simulink library "REC_lib"  (R2015a)
settings: Solver=ode45  StartTime=0.0  StopTime=10.0  RelTol=1e-3
undefined symbols (not defined in the file): REC
libraries: simulink x1, aerolibatmos2 x1
settings Model: Creator=Andrew  LastModifiedBy=Andrew

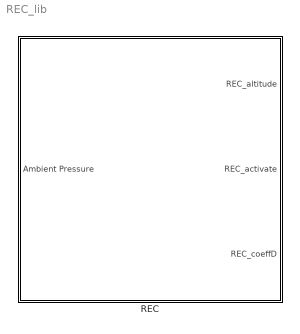
== system REC_lib ==
  REC : Subsystem

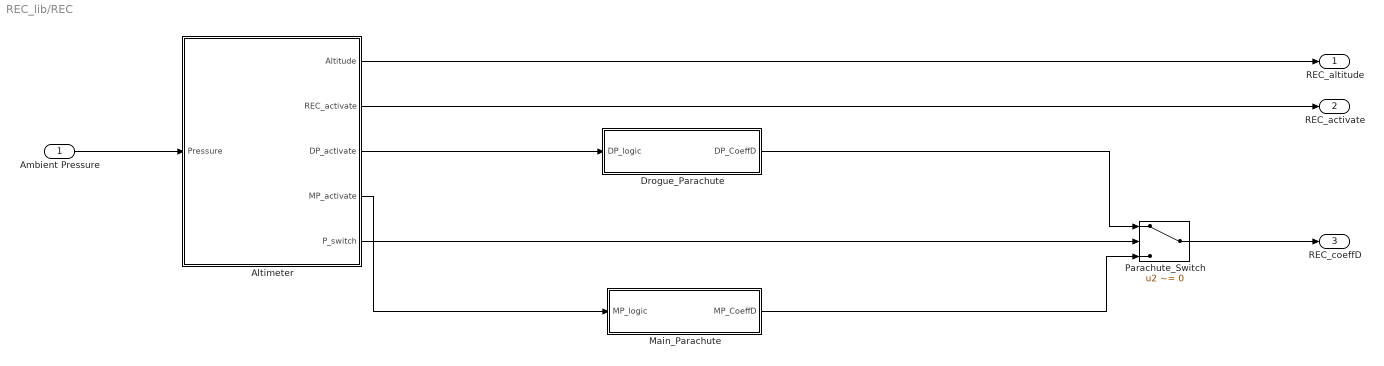
== system REC_lib/REC ==
  Ambient Pressure : Inport
  Altimeter : Subsystem
  Drogue_Parachute : Subsystem
  Main_Parachute : Subsystem
  Parachute_Switch : Switch  Criteria=u2 ~= 0
  REC_altitude : Outport
  REC_activate : Outport  Port=2
  REC_coeffD : Outport  Port=3
  wires:
  Altimeter/4(MP_activate) -> Main_Parachute/1(MP_logic)
  Altimeter/3(DP_activate) -> Drogue_Parachute/1(DP_logic)
  Ambient Pressure/1 -> Altimeter/1(Pressure)
  Altimeter/1(Altitude) -> REC_altitude/1
  Drogue_Parachute/1(DP_CoeffD) -> Parachute_Switch/1
  Main_Parachute/1(MP_CoeffD) -> Parachute_Switch/3
  Altimeter/2(REC_activate) -> REC_activate/1
  Parachute_Switch/1 -> REC_coeffD/1
  Altimeter/5(P_switch) -> Parachute_Switch/2

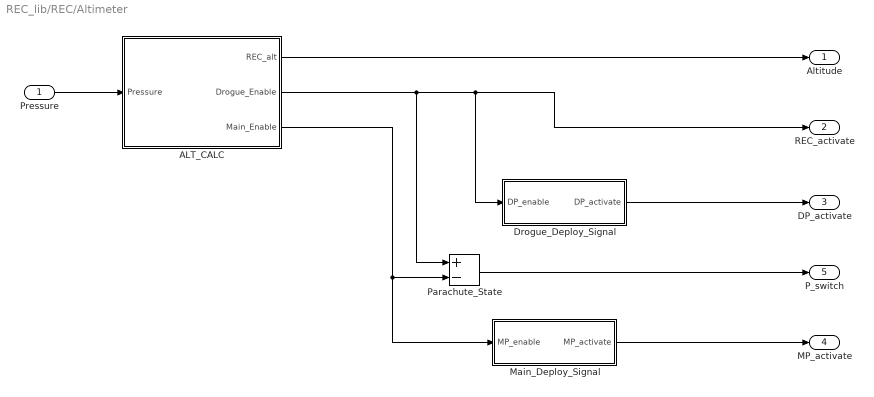
== system REC_lib/REC/Altimeter ==
  Pressure : Inport
  ALT_CALC : Subsystem
  Drogue_Deploy_Signal : Subsystem  TreatAsAtomicUnit=on
  Main_Deploy_Signal : Subsystem  TreatAsAtomicUnit=on
  Parachute_State : Sum  Inputs=+-
  Altitude : Outport
  REC_activate : Outport  Port=2
  DP_activate : Outport  Port=3
  MP_activate : Outport  Port=4
  P_switch : Outport  Port=5
  wires:
  Pressure/1 -> ALT_CALC/1(Pressure)
  ALT_CALC/1(REC_alt) -> Altitude/1
  ALT_CALC/2(Drogue_Enable) -> Parachute_State/1, Drogue_Deploy_Signal/1(DP_enable), REC_activate/1
  ALT_CALC/3(Main_Enable) -> Parachute_State/2, Main_Deploy_Signal/1(MP_enable)
  Drogue_Deploy_Signal/1(DP_activate) -> DP_activate/1
  Main_Deploy_Signal/1(MP_activate) -> MP_activate/1
  Parachute_State/1 -> P_switch/1

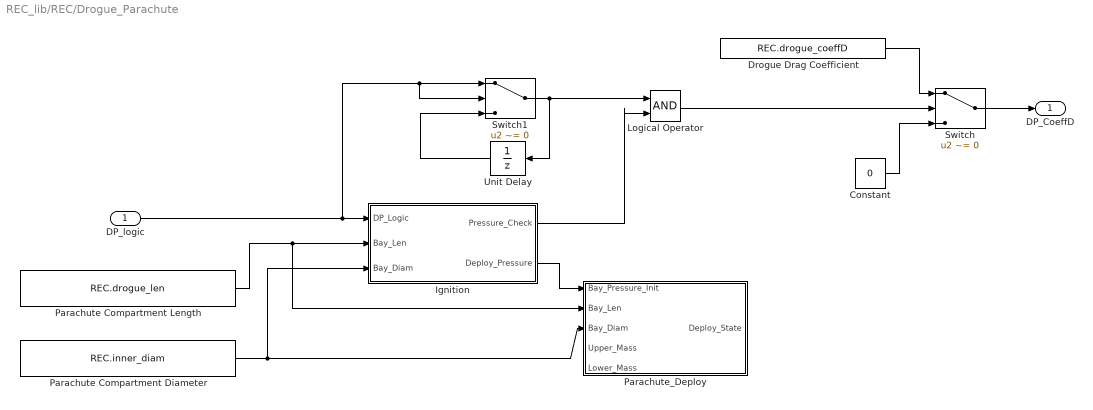
== system REC_lib/REC/Drogue_Parachute ==
  DP_logic : Inport
  Constant : Constant  Value=0
  Drogue Drag Coefficient : FromWorkspace  VariableName=REC.drogue_coeffD  SampleTime=0
  Ignition : Subsystem
  Logical Operator : Logic  AllPortsSameDT=off  OutDataTypeStr=boolean
  Parachute Compartment Diameter : FromWorkspace  VariableName=REC.inner_diam  SampleTime=0
  Parachute Compartment Length : FromWorkspace  VariableName=REC.drogue_len  SampleTime=0
  Parachute_Deploy : Subsystem
  Switch : Switch  Criteria=u2 ~= 0
  Switch1 : Switch  Criteria=u2 ~= 0
  Unit Delay : UnitDelay  SampleTime=-1
  DP_CoeffD : Outport
  wires:
  Switch/1 -> DP_CoeffD/1
  Drogue Drag Coefficient/1 -> Switch/1
  Constant/1 -> Switch/3
  DP_logic/1 -> Switch1/1, Switch1/2, Ignition/1(DP_Logic)
  Unit Delay/1 -> Switch1/3
  Switch1/1 -> Logical Operator/1, Unit Delay/1
  Logical Operator/1 -> Switch/2
  Parachute Compartment Diameter/1 -> Parachute_Deploy/3(Bay_Diam), Ignition/3(Bay_Diam)
  Ignition/1(Pressure_Check) -> Logical Operator/2
  Ignition/2(Deploy_Pressure) -> Parachute_Deploy/1(Bay_Pressure_Init)
  Parachute Compartment Length/1 -> Ignition/2(Bay_Len), Parachute_Deploy/2(Bay_Len)

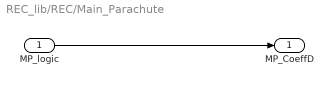
== system REC_lib/REC/Main_Parachute ==
  MP_logic : Inport
  MP_CoeffD : Outport
  wires:
  MP_logic/1 -> MP_CoeffD/1

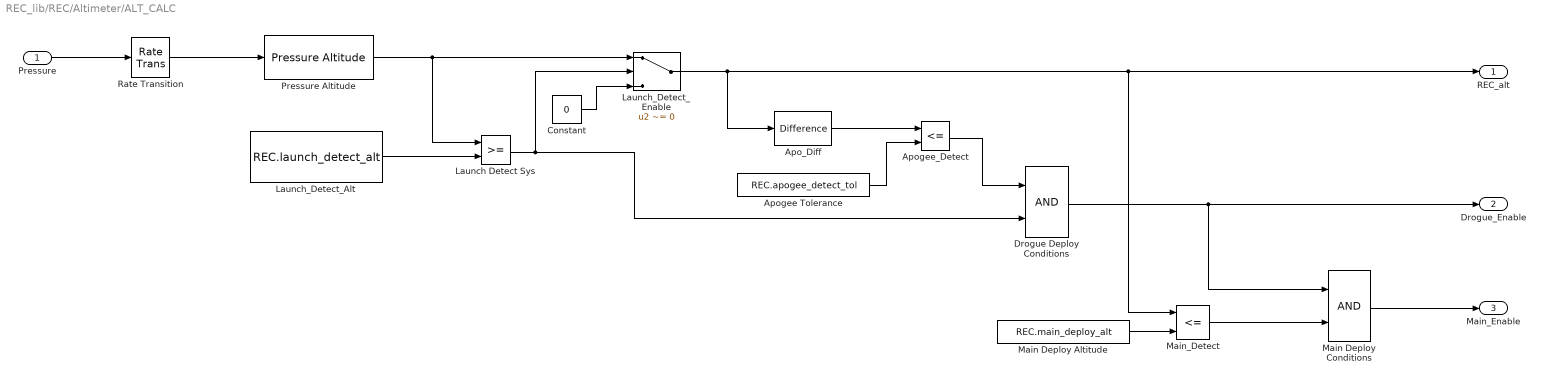
== system REC_lib/REC/Altimeter/ALT_CALC ==
  Pressure : Inport
  Apo_Diff : simulink/Discrete/Difference  ICPrevInput=0.0  InputProcessing=Inherited  OutMin=[]  OutMax=[]  OutDataType=fixdt(1, 16)  OutScaling=2^-10  DoSatur=off
  Apogee Tolerance : FromWorkspace  VariableName=REC.apogee_detect_tol  SampleTime=0
  Apogee_Detect : RelationalOperator  Operator=<=  OutDataTypeStr=boolean
  Constant : Constant  Value=0
  Drogue Deploy Conditions : Logic  AllPortsSameDT=off  OutDataTypeStr=boolean
  Launch Detect Sys : RelationalOperator  OutDataTypeStr=boolean
  Launch_Detect_Alt : FromWorkspace  VariableName=REC.launch_detect_alt  SampleTime=0
  Launch_Detect_Enable : Switch  Criteria=u2 ~= 0
  Main Deploy Altitude : FromWorkspace  VariableName=REC.main_deploy_alt  SampleTime=0
  Main Deploy Conditions : Logic  AllPortsSameDT=off  OutDataTypeStr=boolean
  Main_Detect : RelationalOperator  Operator=<=  OutDataTypeStr=boolean
  Pressure Altitude : aerolibatmos2/Pressure Altitude  units=English  action=Warning
  Rate Transition : RateTransition  OutPortSampleTime=REC.altimeter_sample_time
  REC_alt : Outport
  Drogue_Enable : Outport  Port=2
  Main_Enable : Outport  Port=3
  wires:
  Main Deploy Altitude/1 -> Main_Detect/2
  Apo_Diff/1 -> Apogee_Detect/1
  Pressure/1 -> Rate Transition/1
  Rate Transition/1 -> Pressure Altitude/1
  Apogee Tolerance/1 -> Apogee_Detect/2
  Launch Detect Sys/1 -> Drogue Deploy Conditions/2, Launch_Detect_Enable/2
  Main Deploy Conditions/1 -> Main_Enable/1
  Launch_Detect_Alt/1 -> Launch Detect Sys/2
  Apogee_Detect/1 -> Drogue Deploy Conditions/1
  Constant/1 -> Launch_Detect_Enable/3
  Pressure Altitude/1 -> Launch_Detect_Enable/1, Launch Detect Sys/1
  Launch_Detect_Enable/1 -> Apo_Diff/1, REC_alt/1, Main_Detect/1
  Main_Detect/1 -> Main Deploy Conditions/2
  Drogue Deploy Conditions/1 -> Drogue_Enable/1, Main Deploy Conditions/1

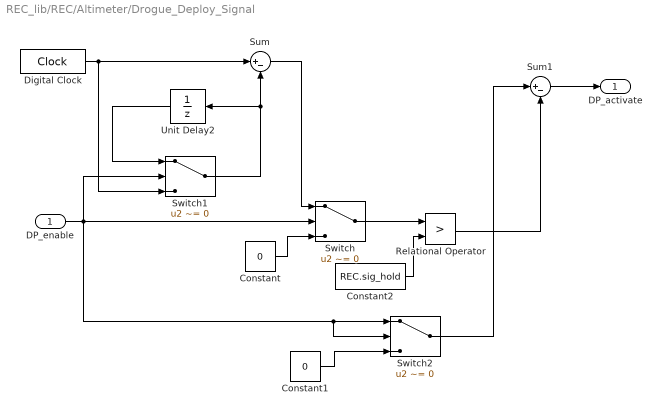
== system REC_lib/REC/Altimeter/Drogue_Deploy_Signal ==
  DP_enable : Inport
  Constant : Constant  Value=0
  Constant1 : Constant  Value=0
  Constant2 : Constant  Value=REC.sig_hold
  Digital Clock : DigitalClock  SampleTime=0.0025
  Relational Operator : RelationalOperator  Operator=>  OutDataTypeStr=boolean
  Sum : Sum  Inputs=|+-
  Sum1 : Sum  Inputs=|+-
  Switch : Switch  Criteria=u2 ~= 0
  Switch1 : Switch  Criteria=u2 ~= 0
  Switch2 : Switch  Criteria=u2 ~= 0
  Unit Delay2 : UnitDelay  SampleTime=-1
  DP_activate : Outport
  wires:
  Constant/1 -> Switch/3
  Digital Clock/1 -> Sum/1, Switch1/3
  Sum/1 -> Switch/1
  Switch/1 -> Relational Operator/1
  Switch1/1 -> Unit Delay2/1, Sum/2
  Unit Delay2/1 -> Switch1/1
  DP_enable/1 -> Switch2/1, Switch2/2, Switch1/2, Switch/2
  Constant1/1 -> Switch2/3
  Sum1/1 -> DP_activate/1
  Switch2/1 -> Sum1/1
  Relational Operator/1 -> Sum1/2
  Constant2/1 -> Relational Operator/2

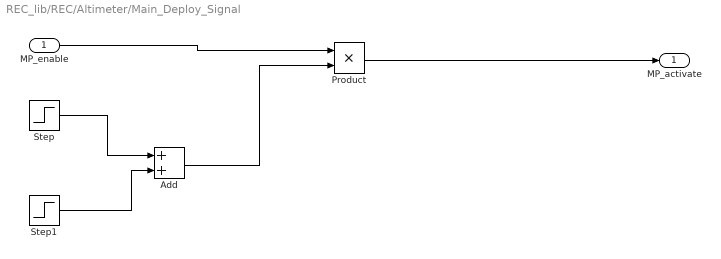
== system REC_lib/REC/Altimeter/Main_Deploy_Signal ==
  MP_enable : Inport
  Add : Sum
  Product : Product
  Step : Step  Time=0  SampleTime=0
  Step1 : Step  After=-1  SampleTime=0
  MP_activate : Outport
  wires:
  Product/1 -> MP_activate/1
  MP_enable/1 -> Product/1
  Step/1 -> Add/1
  Step1/1 -> Add/2
  Add/1 -> Product/2

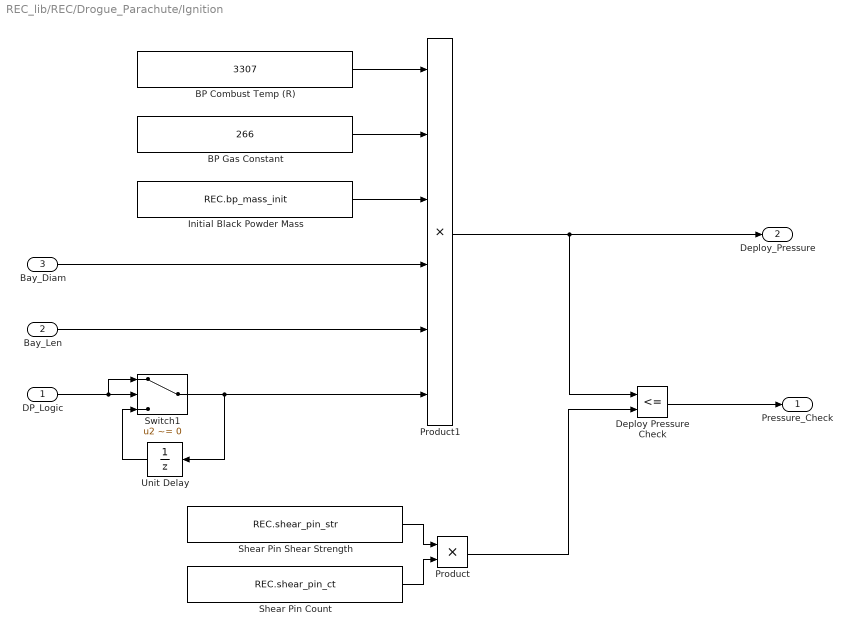
== system REC_lib/REC/Drogue_Parachute/Ignition ==
  DP_Logic : Inport
  Bay_Len : Inport  Port=2
  Bay_Diam : Inport  Port=3
  BP Combust Temp (R) : FromWorkspace  VariableName=3307  SampleTime=0
  BP Gas Constant : FromWorkspace  VariableName=266  SampleTime=0
  Deploy Pressure Check : RelationalOperator  Operator=<=  OutDataTypeStr=boolean
  Initial Black Powder Mass : FromWorkspace  VariableName=REC.bp_mass_init  SampleTime=0
  Product : Product
  Product1 : Product  Inputs=6
  Shear Pin Count : FromWorkspace  VariableName=REC.shear_pin_ct  SampleTime=0
  Shear Pin Shear Strength : FromWorkspace  VariableName=REC.shear_pin_str  SampleTime=0
  Switch1 : Switch  Criteria=u2 ~= 0
  Unit Delay : UnitDelay  SampleTime=-1
  Pressure_Check : Outport
  Deploy_Pressure : Outport  Port=2
  wires:
  BP Combust Temp (R)/1 -> Product1/1
  Product/1 -> Deploy Pressure Check/2
  Shear Pin Shear Strength/1 -> Product/1
  BP Gas Constant/1 -> Product1/2
  Shear Pin Count/1 -> Product/2
  Deploy Pressure Check/1 -> Pressure_Check/1
  Switch1/1 -> Unit Delay/1, Product1/6
  Product1/1 -> Deploy Pressure Check/1, Deploy_Pressure/1
  Initial Black Powder Mass/1 -> Product1/3
  Unit Delay/1 -> Switch1/3
  DP_Logic/1 -> Switch1/1, Switch1/2
  Bay_Diam/1 -> Product1/4
  Bay_Len/1 -> Product1/5

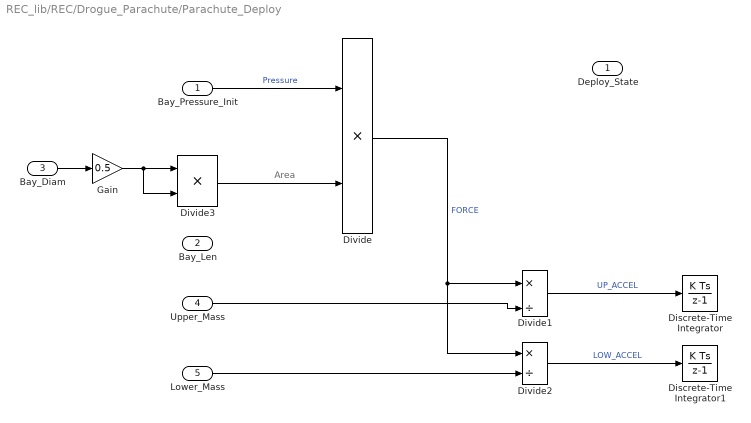
== system REC_lib/REC/Drogue_Parachute/Parachute_Deploy ==
  note: Area
  Bay_Pressure_Init : Inport
  Bay_Len : Inport  Port=2
  Bay_Diam : Inport  Port=3
  Upper_Mass : Inport  Port=4
  Lower_Mass : Inport  Port=5
  Discrete-Time Integrator : DiscreteIntegrator  InitialConditionSetting=State (most efficient)
  Discrete-Time Integrator1 : DiscreteIntegrator  InitialConditionSetting=State (most efficient)
  Divide : Product  Inputs=**
  Divide1 : Product  Inputs=*/
  Divide2 : Product  Inputs=*/
  Divide3 : Product  Inputs=**
  Gain : Gain  Gain=0.5
  Deploy_State : Outport
  wires:
  Bay_Pressure_Init/1 -> Divide/1  "Pressure"
  Bay_Diam/1 -> Gain/1
  Upper_Mass/1 -> Divide1/2
  Divide/1 -> Divide2/1, Divide1/1  "FORCE"
  Lower_Mass/1 -> Divide2/2
  Divide2/1 -> Discrete-Time Integrator1/1  "LOW_ACCEL"
  Divide1/1 -> Discrete-Time Integrator/1  "UP_ACCEL"
  Divide3/1 -> Divide/2
  Gain/1 -> Divide3/2, Divide3/1
